simulink model "AC_gen_MGES"  (R2025a)
settings: Solver=VariableStepAuto  StartTime=0.0  StopTime=10.0  RelTol=1e-3
undefined symbols (not defined in the file): buses_lf, gen_static_params, Grid_op_MGES, Grid_op_SG, Matrix_flux_to_i, Ps_lf, Sb, SGs_nodes
(part 1 of 2)
settings Model: Creator=atomas  LastModifiedBy=atomas

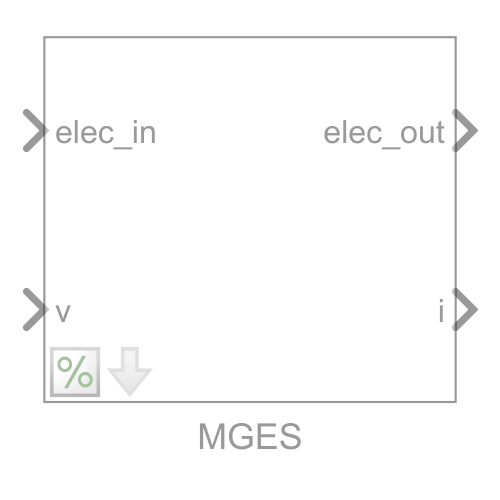
[thumbnail: Simulink's stored preview of the top-level diagram]
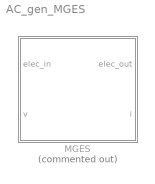
== system AC_gen_MGES ==
  MGES : Subsystem  Commented=on  mask(Synchronous machine){SGs_nodes=SGs_nodes, FBASE=50, D=0, H=3, Psimag_pu=0.8, Lssd_pu=0.1, Lssq_pu=0.1, Rs_pu=0.001, Lmd_pu=0.1, Lmq_pu=0.1, Rfd_pu=0.01, Lfd_pu=0.1, Rkd1_pu=1e6, Lkd1_pu=1e6, Rkd2_pu=1e6, Lkd2_pu=1e6, Rkq1_pu=1e6, Lkq1_pu=1e6, Rkq2_pu=1e6, Lkq2_pu=1e6, Rkq3_pu=1e6, Lkq3_pu=1e6, T_e=1, T_v=1, T_1=1, T_2=1, K_A=1, K_C=0, K_P=0, K_PR=1, K_IR=1, K_PM=1, K_IM=1, R_p=0.05, T_1g=1, T_2g=1, T_3=1, T_4=1, T_5=1, T_6=1, K_1=0, K_3=0, K_5=0, T_w1=1, T_w2=1, T_9=1, M=1, K_S1=0, T_1p=1, T_2p=1, T_3p=1, T_4p=1, T_7p=1, K_S2=1, K_S3=1}
      mask prompts: FBASE "Base frequency (Hz)"; D "Damping (pu)"; H "Inertia (s)"; Psimag_pu "Permanent flux (pu)"; Lssd_pu "Stator inductances (pu) Ld"; Lssq_pu "Stator inductances (pu) Lq"; Rs_pu "Stator resistances (pu)"; Lmd_pu "d-axis mutual inductance (pu)"; Lmq_pu "q-axis mutual inductance (pu)"; Rfd_pu "Excitation resistance (pu)"; Lfd_pu "Excitation inductance (pu)"; Rkd1_pu "d-axis damper resistance 1 (pu)"; Lkd1_pu "d-axis damper inductance 1 (pu)"; Rkd2_pu "d-axis damper resistance 2 (pu)"; Lkd2_pu "d-axis damper inductance 2 (pu)"; Rkq1_pu "q-axis damper resistance 1 (pu)"; Lkq1_pu "q-axis damper inductance 1 (pu)"; Rkq2_pu "q-axis damper resistance 2 (pu)"; Lkq2_pu "q-axis damper inductance 2 (pu)"; Rkq3_pu "q-axis damper resistance 3 (pu)"; Lkq3_pu "q-axis damper inductance 3 (pu)"; T_1p "T_1"
      mask help: Synchronous machine modelled in d-q reference frame.
      mask init:
      | mdlWks = get_param(bdroot,'ModelWorkspace'); % Get the model workspace
      | block_name = get_param(gcb,'Name');
      | try
      |     bvarname = get_param(get_param(get_param(...
      |         gcb, 'Parent'), 'Parent'), 'bvarname');
      |     block_buses = mdlWks.getVariable([bvarname block_name 's_buses']);
      | 	block_idx = mdlWks.getVariable([bvarname block_name '_idx']);
      |     block_toM = mdlWks.getVariable([bvarname block_name 's_toM']);
      |     fref = mdlWks.getVariable([bvarname 'fref']);
      |     block_fref = fref.(block_name);
      | catch ME % block in initialisation
      |     %errordlg(ME.message)
      |     try
      |         block_buses = 1:length(mdlWks.getVariable([block_name 's_buses']));
      | 	    block_idx = mdlWks.getVariable([block_name '_idx']);
      |         block_toM = mdlWks.getVariable([block_name 's_toM']);
      |         fref = mdlWks.getVariable('fref');
      | 	    block_fref = fref.(block_name);
      |     catch ME
      |         %errordlg(ME.message)
      |     end
      | end
      | 
      |     
      |     n = length(block_buses);
      |     Lbiginv = zeros(9*n,9*n);
      |     if isscalar(Lssd_pu)
      |         Lssd_pu = Lssd_pu*ones(1, n);
      |     end
      |     if isscalar(Lssq_pu)
      |         Lssq_pu = Lssq_pu*ones(1, n);
      |     end
      |     if isscalar(Lmd_pu)
      |         Lmd_pu = Lmd_pu*ones(1, n);
      |     end
      |     if isscalar(Lmq_pu)
      |         Lmq_pu = Lmq_pu*ones(1, n);
      |     end
      |     if isscalar(Lfd_pu)
      |         Lfd_pu = Lfd_pu*ones(1, n);
      |     end
      |     if isscalar(Lssd_pu)
      |         Lssd_pu = Lssd_pu*ones(1, n);
      |     end
      |     if isscalar(Lkd1_pu)
      |         Lkd1_pu = Lkd1_pu*ones(1, n);
      |     end
      |     if isscalar(Lkd2_pu)
      |         Lkd2_pu = Lkd2_pu*ones(1, n);
      |     end
      |     if isscalar(Lkq1_pu)
      |         Lkq1_pu = Lkq1_pu*ones(1, n);
      |     end
      |     if isscalar(Lkq2_pu)
      |         Lkq2_pu = Lkq2_pu*ones(1, n);
      |     end
      |     if isscalar(Lkq3_pu)
      |         Lkq3_pu = Lkq3_pu*ones(1, n);
      |     end
      |     for i=1:n
      |         j = 9*(i-1)+1;
      |         Ldq0 = [Lssd_pu(i), 0 0; 0, Lssq_pu(i), 0; 0, 0, 0.0001]; 
      |         Ladq0 = [Lmd_pu(i), Lmd_pu(i), Lmd_pu(i), 0 0 0; 0, 0, 0, Lmq_pu(i), Lmq_pu(i), Lmq_pu(i); zeros(1, 6)];
      |         Lk = [Lmd_pu(i)*ones(3,3), zeros(3,3); zeros(3,3), Lmq_pu(i)*ones(3,3)] +...
      |             diag([Lfd_pu(i), Lkd1_pu(i), Lkd2_pu(i), Lkq1_pu(i), Lkq2_pu(i), Lkq3_pu(i)]);
      |         L = [-Ldq0, Ladq0; -Ladq0', Lk];
      |         Lbiginv(j:(j+8), j:(j+8)) = inv(L);
      |     end
      | 
      |     if isscalar(K_C)
      |         K_C = K_C*ones(1, n);
      |     end
      |     if isscalar(K_P)
      |         K_P = K_P*ones(1, n);
      |     end
      |     if isscalar(T_1)
      |         T_1 = T_1*ones(1, n);
      |     end
      |     if isscalar(T_2)
      |         T_2 = T_2*ones(1, n);
      |     end
      mask Help: web([extractBefore(get_param(bdroot, 'filename'),gcs) 'Documentation/SM.html'])
      mask DialogControl Params Prompt: Parameters
      mask DialogControl AVR Prompt: AVR
      mask DialogControl Gov Prompt: Speed governor
      mask DialogControl PSS Prompt: Power system stabiliser

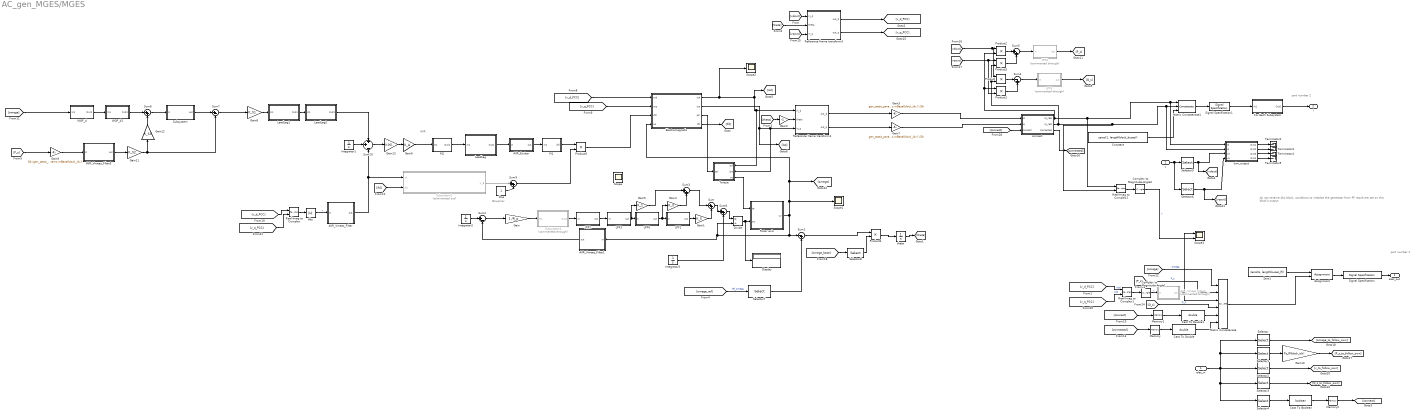
== system AC_gen_MGES/MGES ==
  note: AVR
  note: port number 2
  note: port number 1
  note: do not rename this block, conditions to initialise the generator from PF result are set on this block's output
  note: Governor
  elec_in : Inport
  v : Inport  Port=2
  AVR_Exciter : Subsystem  mask{T_s=T_e}
      mask prompts: T_s "Filter time constant"
  AVR_Vmeas_Filter : Subsystem  mask{T_r=T_v}
      mask prompts: T_r "Filter time constant"
  AVR_Vmeas_Filter1 : Subsystem  mask{T_r=0.01}
      mask prompts: T_r "Filter time constant"
  AVR_Vmeas_Filter2 : Subsystem  Commented=through  mask{T_r=0.01}
      mask prompts: T_r "Filter time constant"
      mask Display:
      | try
      |     dpoly(1, [T_r, 1])
      | catch
      | end
  AVR_Vmeas_Filter3 : Subsystem  mask{T_r=T_7p}
      mask prompts: T_r "Filter time constant"
  Abs : Abs  SaturateOnIntegerOverflow=off
  Assignment : Assignment  NumberOfDimensions=2  DiagnosticForDimensions=Warning  IndexOptions=Assign all,Index vector (dialog)  Indices=1,block_idx  OutputSizes=1,1
  Cast To Boolean : DataTypeConversion  OutDataTypeStr=boolean  SaturateOnIntegerOverflow=off  RndMeth=Floor
  Cast To Double : DataTypeConversion  OutDataTypeStr=double  SaturateOnIntegerOverflow=off  RndMeth=Floor
  Cast To Double1 : DataTypeConversion  OutDataTypeStr=double  SaturateOnIntegerOverflow=off  RndMeth=Floor
  Complex to Magnitude-Angle1 : ComplexToMagnitudeAngle  Output=Magnitude
  Complex to Magnitude-Angle2 : ComplexToMagnitudeAngle  Output=Magnitude
  Constant : Constant  Value=zeros(1, length(block_buses))  VectorParams1D=off
  Display : Display
  Divide : Product  Inputs=*/
  Electromagnetic : Subsystem  Variant=on  VariantControlMode=label  LabelModeActiveChoice=order 8
  For Each Subsystem : Subsystem  TreatAsAtomicUnit=on
  Gain : Gain  Gain=1./R_p
  Gain1 : Gain  Gain=K_5
  Gain10 : Gain  Gain=Ps_lf(block_idx)
  Gain11 : Gain  Gain=K_S2
  Gain12 : Gain  Gain=K_S3
  Gain13 : Gain  Gain=0.001
  Gain2 : Gain  Gain=-1
  Gain3 : Gain  Gain=gen_static_params.mBase(block_idx)'./Sb
  Gain4 : Gain  Gain=K_3
  Gain5 : Gain  Gain=K_1
  Gain6 : Gain  Gain=K_A
  Gain7 : Gain  Gain=gen_static_params.mBase(block_idx)'./Sb
  Gain8 : Gain  Gain=K_S1
  Gain9 : Gain  Gain=Sb./gen_static_params.mBase(block_idx)'
  Integrator1 : Integrator  InitialCondition=Grid_op_MGES.op.States(13).x'
  Integrator2 : Integrator  InitialCondition=Grid_op_MGES.op.States(14).x'
  Integrator3 : Integrator  InitialCondition=Grid_op_MGES.op.States(15).x'
  LPF1 : Subsystem  mask{T_s=T_6}
      mask prompts: T_s "Filter time constant"
  LPF2 : Subsystem  mask{T_s=T_3}
      mask prompts: T_s "Filter time constant"
  LPF3 : Subsystem  mask{T_s=T_4}
      mask prompts: T_s "Filter time constant"
  LPF4 : Subsystem  Commented=through  mask{T_s=0.01}
      mask prompts: T_s "Filter time constant"
      mask Display:
      | try
      |     dpoly(1, [T_s, 1])
      | catch
      | end
  LPF5 : Subsystem  Commented=through  mask{T_s=0.01}
      mask prompts: T_s "Filter time constant"
      mask Display:
      | try
      |     dpoly(1, [T_s, 1])
      | catch
      | end
  LPF6 : Subsystem  mask{T_s=T_5}
      mask prompts: T_s "Filter time constant"
  LeadLag : Subsystem
  LeadLag1 : Subsystem  mask{T_2=T_1p, T_1=T_2p}
      mask help:
      | Transfer function:
      |
      |   1 + sT_2
      | ---------------
      |   1 + sT_1
  LeadLag2 : Subsystem  mask{T_2=T_3p, T_1=T_4p}
      mask help:
      | Transfer function:
      |
      |   1 + sT_2
      | ---------------
      |   1 + sT_1
  Matrix Concatenate : Concatenate  NumInputs=6  Mode=Multidimensional array
  Matrix Concatenate1 : Concatenate  NumInputs=3  Mode=Multidimensional array
  Memory : Memory  InitialCondition=1
  Memory1 : Memory  InitialCondition=1
  Memory2 : Memory  InitialCondition=1
  One : Constant  OutDataTypeStr=Inherit: Inherit via back propagation
  PI1 : Subsystem
  PI2 : Subsystem
  Product{,1..5} (6 alike) : Product
  Real-Imag to Complex : RealImagToComplex
  Real-Imag to Complex1 : RealImagToComplex
  Real-Imag to Complex2 : RealImagToComplex
  Reference frame transform1 : Subsystem
  Reference frame transform3 : Subsystem
  Rotor axis : Subsystem
  Scope : Scope
      settings: ActiveDisplayYMinimum=-1  ActiveDisplayYMaximum=1  DataLoggingVariableName=ScopeData13
  Scope1 : Scope
      settings: ActiveDisplayYMinimum=-0.058141408811601208  ActiveDisplayYMaximum=2.1702525958532117  DataLoggingVariableName=ScopeData3
  Scope2 : Scope
      settings: ActiveDisplayYMinimum=-0.402690614368146  ActiveDisplayYMaximum=1.3038964261892889  DataLoggingVariableName=ScopeData9
  Scope3 : Scope  NumInputPorts=2
      settings: ActiveDisplayYMinimum=0.29123  ActiveDisplayYMaximum=1.9416  DataLoggingVariableName=ScopeData3
  Selector : Selector  NumberOfDimensions=2  InputPortWidth=3  IndexOptions=Index vector (dialog),Index vector (dialog)  Indices=1,block_idx  OutputSizes=1,1
  Selector1 : Selector  NumberOfDimensions=2  InputPortWidth=3  IndexOptions=Index vector (dialog),Index vector (dialog)  Indices=2,block_idx  OutputSizes=1,1
  Selector2 : Selector  NumberOfDimensions=2  InputPortWidth=3  IndexOptions=Index vector (dialog),Index vector (dialog)  Indices=3,block_idx  OutputSizes=1,1
  Selector3 : Selector  NumberOfDimensions=2  InputPortWidth=3  IndexOptions=Index vector (dialog),Index vector (dialog)  Indices=4,block_idx  OutputSizes=1,1
  Selector4 : Selector  NumberOfDimensions=2  InputPortWidth=3  IndexOptions=Index vector (dialog),Index vector (dialog)  Indices=5,block_idx  OutputSizes=1,1
  Selector5 : Selector  NumberOfDimensions=2  InputPortWidth=3  IndexOptions=Index vector (dialog),Index vector (dialog)  Indices=1,block_buses  OutputSizes=1,1
  Selector6 : Selector  NumberOfDimensions=2  InputPortWidth=3  IndexOptions=Index vector (dialog),Index vector (dialog)  Indices=2,block_buses  OutputSizes=1,1
  Selector7 : Selector  InputPortWidth=length(fref.ref_units)  IndexOptions=Index vector (dialog)  Indices=block_fref  OutputSizes=1
  Selector8 : Selector  InputPortWidth=length(fref.ref_units)  IndexOptions=Index vector (dialog)  Indices=block_fref  OutputSizes=1
  Signal Specification : SignalSpecification  Dimensions=[6 length(buses_lf)]
  Signal Specification1 : SignalSpecification  Dimensions=[3 length(block_buses)]
  Subsystem : Subsystem
  Subsystem1 : Subsystem  Commented=on  mask{K_P=K_P}
      mask init:
      | if all(K_P == 0)
      |         set_param(gcb, 'Commented', 'on')
      |     else
      |         set_param(gcb, 'Commented', 'off')
      |     end
  Subsystem4 : Subsystem  Commented=through  mask{T_2=T_2, T_1=T_1}
      mask help:
      | Transfer function:
      |
      |   1 + sT_2
      | ---------------
      |   1 + sT_1
  Sum{,3,5..6,8..9} (6 alike) : Sum  Inputs=|++
  Sum1 : Sum  Inputs=|-+
  Sum10 : Sum  Inputs=+|+|-
  Sum2 : Sum  Inputs=|+-
  Sum4 : Sum  Inputs=|-+
  Sum7 : Sum  Inputs=|+-
  Terminator{2..5} (4 alike) : Terminator
  Torque : Subsystem
      settings: PortSchema="{\"entries\":[{\"content\":{\"sides\":[{\"content\":{\"connectorIds\":[\"In1\"]},\"type\":\"ConnectorPlacement.EquallySpacedRectSide\",\"uuid\":\"b7abd3bc-22dd-4669-aa40-98bc76884565\"},{\"content\":{\"connectorIds\":[\"In2\",\"In3\",\"Out1\"],\"side\":\"RIGHT\"},\"type\":\"ConnectorPlacement.EquallySpacedRectSide\",\"uuid\":\"e9abb552-b46d-48ed-aa1f-0e9dac604fea\"},{\"content\":{\"connectorIds\":[],\"side\":\"TOP\"},\"type\":\"ConnectorPlacement.EquallySpacedRectSide\",\"uuid\":\"4b14997d-8f32-4cfb-8a1b-18cffb093d28\"}]},\"type\":\"ConnectorPlacement.EquallySpacedConnector\",\"uuid\":\"d6624493-e930-4f0d-8cbe-17f96cb72edc\"}],\"packageUris\":[\"http://schema.mathworks.com/mf0/Connector/R2020b\"],\"version\":\"1.0\"}"
  WOF_d : Subsystem
  WOF_d1 : Subsystem
  Zero1 : Constant  Value=zeros(6, length(buses_lf))  VectorParams1D=off  OutDataTypeStr=Inherit: Inherit via back propagation
  connect : Subsystem
  theta : Integrator  InitialCondition=Grid_op_MGES.op.States(33).x'  UpperSaturationLimit=2*pi  LowerSaturationLimit=0
  trim_output : Subsystem
  elec_out : Outport
  i : Outport  Port=2
  wires:
  One/1 -> Sum9/2
  Sum9/1 -> Product5/2
  Subsystem1/1(V_B) -> Sum9/1
  Product5/1 -> Electromagnetic/3(vfd)
  Divide/1 -> Rotor axis/2(tm), Display/1
  LeadLag2/1(Out1) -> Sum10/1
  Gain9/1 -> AVR_Vmeas_Filter3/1(in)
  Integrator3/1 -> Sum8/2
  Sum8/1 -> Divide/1
  Sum/1 -> Sum8/1
  Gain13/1 -> Gain6/1
  Sum10/1 -> Gain13/1
  Torque/1(te) -> Rotor axis/1(te)
  Integrator2/1 -> Sum2/1
  [P_s] -> Gain9/1
  AVR_Vmeas_Filter3/1(out) -> Gain11/1
  Gain11/1 -> Gain12/1, Sum7/2
  Gain12/1 -> Sum6/2
  Sum7/1 -> Gain8/1
  Subsystem/1(out) -> Sum7/1
  Sum6/1 -> Subsystem/1(in)
  WOF_d1/1(Out1) -> Sum6/1
  [omega] -> WOF_d/1(In1)
  LeadLag1/1(Out1) -> LeadLag2/1(In1)
  Gain8/1 -> LeadLag1/1(In1)
  WOF_d/1(Out1) -> WOF_d1/1(In1)
  Gain7/1 -> connect/2(iq)
  Gain3/1 -> connect/1(id)
  Gain5/1 -> Sum3/1
  Gain4/1 -> Sum3/2
  Sum3/1 -> Sum/1
  Rotor axis/1(wr) -> AVR_Vmeas_Filter1/1(in), Divide/2, Sum1/1, Scope1/1, [omega], Electromagnetic/4(ws)
  Gain1/1 -> Sum/2
  LPF1/1(out) -> Gain1/1
  LPF3/1(out) -> LPF6/1(in), Gain5/1
  PI1/1(vfd) -> Product5/1
  [ifd] -> Subsystem1/2(ifd)
  AVR_Exciter/1(out) -> PI1/1(In1)
  PI2/1(Out1) -> LeadLag/1(In1)
  Electromagnetic/4(ifd) -> [ifd]
  Electromagnetic/3(psi) -> Torque/1(psi)
  [v_q_PCC] -> Electromagnetic/2(vsq)
  [v_d_PCC] -> Electromagnetic/1(vsd)
  Electromagnetic/1(isd) -> [isd], Torque/2(isd), Reference frame transform1/1(in_d), Scope2/1
  Electromagnetic/2(isq) -> Reference frame transform1/3(in_q), Torque/3(isq), [isq]
  Complex to Magnitude-Angle2/1 -> Scope3/2  "v"
  Real-Imag to Complex2/1 -> Complex to Magnitude-Angle2/1
  AVR_Vmeas_Filter2/1(out) -> Scope3/1, Matrix Concatenate/3
  AVR_Vmeas_Filter1/1(out) -> Sum2/2
  Real-Imag to Complex/1 -> Abs/1
  [v_q_PCC] -> Real-Imag to Complex/2
  Abs/1 -> AVR_Vmeas_Filter/1(in)  "v"
  [v_d_PCC] -> Real-Imag to Complex/1
  LeadLag/1(Out1) -> AVR_Exciter/1(in)
  AVR_Vmeas_Filter/1(out) -> Subsystem1/1(vt), Sum10/3
  Gain6/1 -> PI2/1(In1)
  Integrator1/1 -> Sum10/2
  Sum2/1 -> Gain/1
  Gain/1 -> Subsystem4/1(In1)
  Sum1/1 -> Product4/1
  Product4/1 -> theta/1
  [omega_base] -> Selector8/1
  Selector8/1 -> Product4/2
  Selector7/1 -> Sum1/2
  Memory2/1 -> [connect]
  Memory1/1 -> Cast To Double1/1
  Gain10/1 -> [P_s_to_follow_own]
  Memory/1 -> Cast To Double/1
  Reference frame transform3/2(out_q) -> [v_q_PCC]
  Reference frame transform3/1(out_d) -> [v_d_PCC]
  [vdout] -> Reference frame transform3/1(in_d)
  [vqout] -> Reference frame transform3/3(in_q)
  Selector6/1 -> trim_output/4(vq), [vqout]
  Selector5/1 -> trim_output/3(vd), [vdout]
  v/1 -> Selector5/1, Selector6/1
  trim_output/2(Out2) -> Terminator3/1
  trim_output/4(Out4) -> Terminator5/1
  trim_output/1(Out1) -> Terminator2/1
  trim_output/3(Out3) -> Terminator4/1
  connect/2(iq_real) -> Matrix Concatenate1/2, trim_output/2(iq), Real-Imag to Complex2/2, Product/2, Product3/2
  For Each Subsystem/1(Out1) -> i/1
  Constant/1 -> Matrix Concatenate1/3
  Signal Specification1/1 -> For Each Subsystem/1(In1)
  Matrix Concatenate1/1 -> Signal Specification1/1
  Matrix Concatenate/1 -> Assignment/2
  Assignment/1 -> Signal Specification/1
  elec_in/1 -> Selector/1, Selector1/1, Selector2/1, Selector3/1, Selector4/1
  Signal Specification/1 -> elec_out/1
  Zero1/1 -> Assignment/1
  Cast To Boolean/1 -> Memory2/1
  Selector4/1 -> Cast To Boolean/1
  connect/1(id_real) -> Product2/2, Product1/1, Matrix Concatenate1/1, trim_output/1(id), Real-Imag to Complex2/1
  [connect] -> connect/3(connect)
  connect/3(connected) -> [connected]
  [v_q_PCC] -> Real-Imag to Complex1/2  "voq"
  [v_d_PCC] -> Real-Imag to Complex1/1  "vod"
  [vqout] -> Product1/2, Product3/1
  [vdout] -> Product2/1, Product/1
  Real-Imag to Complex1/1 -> Complex to Magnitude-Angle1/1
  Cast To Double/1 -> Matrix Concatenate/6
  Cast To Double1/1 -> Matrix Concatenate/5
  [connected] -> Memory/1
  [connect] -> Memory1/1
  Selector2/1 -> [v_to_follow_own]
  Selector1/1 -> Gain10/1
  Selector/1 -> [omega_to_follow_own]
  Selector3/1 -> [Q_s_to_follow_own]
  [Q_s] -> Matrix Concatenate/4  "Q_s"
  Complex to Magnitude-Angle1/1 -> AVR_Vmeas_Filter2/1(in)  "v"
  [omega] -> Matrix Concatenate/1  "omega"
  [P_s] -> Matrix Concatenate/2  "P_s"
  LPF4/1(out) -> [P_s]
  Subsystem4/1(Out1) -> LPF2/1(in)
  Reference frame transform1/1(out_d) -> Gain3/1
  Product2/1 -> Sum5/1
  [omega_ref] -> Selector7/1  "ref_omega"
  Product3/1 -> Sum5/2
  Sum5/1 -> LPF4/1(in)
  Sum4/1 -> LPF5/1(in)
  LPF2/1(out) -> LPF3/1(in)
  [theta] -> Gain2/1
  LPF6/1(out) -> LPF1/1(in), Gain4/1
  [theta] -> Reference frame transform3/2(theta)
  Gain2/1 -> Reference frame transform1/2(theta)
  theta/1 -> [theta]
  Product1/1 -> Sum4/2
  Product/1 -> Sum4/1
  Reference frame transform1/2(out_q) -> Gain7/1
  LPF5/1(out) -> [Q_s]

== system AC_gen_MGES/MGES/AVR_Exciter ==
  in : Inport
  Gain : Gain  Gain=1./T_s
  Sum4 : Sum  Inputs=|+-
  x_a : Integrator  InitialCondition=Grid_op_MGES.op.States(1).x'
  out : Outport
  wires:
  x_a/1 -> Sum4/2, out/1
  in/1 -> Sum4/1
  Sum4/1 -> Gain/1
  Gain/1 -> x_a/1

== system AC_gen_MGES/MGES/AVR_Vmeas_Filter ==
  in : Inport
  Gain : Gain  Gain=1./T_r
  Sum4 : Sum  Inputs=|+-
  x_a : Integrator  InitialCondition=Grid_op_MGES.op.States(2).x'
  out : Outport
  wires:
  x_a/1 -> Sum4/2, out/1
  in/1 -> Sum4/1
  Sum4/1 -> Gain/1
  Gain/1 -> x_a/1

== system AC_gen_MGES/MGES/AVR_Vmeas_Filter1 ==
  in : Inport
  Gain : Gain  Gain=1/T_r
  Sum4 : Sum  Inputs=|+-
  x_a : Integrator  InitialConditionSource=external  InitialCondition=Grid_op_MGES.op.States(3).x'
  out : Outport
  wires:
  Gain/1 -> x_a/1
  Sum4/1 -> Gain/1
  in/1 -> Sum4/1, x_a/2
  x_a/1 -> out/1, Sum4/2

== system AC_gen_MGES/MGES/AVR_Vmeas_Filter2 ==
  in : Inport
  Gain : Gain  Gain=1/T_r
  Sum4 : Sum  Inputs=|+-
  x_a : Integrator  InitialCondition=Grid_op_SG.op.States(5).x'
  out : Outport
  wires:
  x_a/1 -> Sum4/2, out/1
  in/1 -> Sum4/1
  Sum4/1 -> Gain/1
  Gain/1 -> x_a/1

== system AC_gen_MGES/MGES/AVR_Vmeas_Filter3 ==
  in : Inport
  Gain : Gain  Gain=1./T_r
  Sum4 : Sum  Inputs=|+-
  x_a : Integrator  InitialCondition=Grid_op_MGES.op.States(4).x'
  out : Outport
  wires:
  Gain/1 -> x_a/1
  Sum4/1 -> Gain/1
  in/1 -> Sum4/1
  x_a/1 -> out/1, Sum4/2

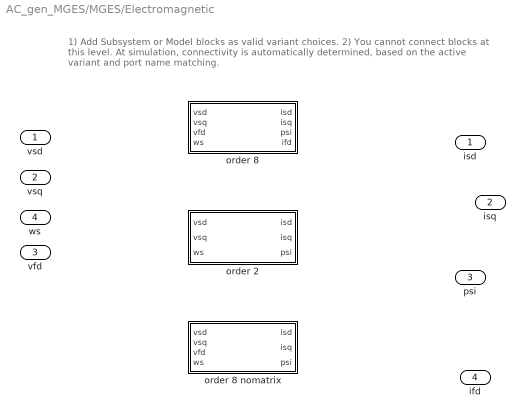
== system AC_gen_MGES/MGES/Electromagnetic ==
  note: 1) Add Subsystem or Model blocks as valid variant choices.
      | 2) You cannot connect blocks at this level. At simulation, connectivity is automatically
      | determined, based on the active variant and port name matching.
  vsd : Inport
  vsq : Inport  Port=2
  vfd : Inport  Port=3
  ws : Inport  Port=4
  order 2 : Subsystem  VariantControl=order 2
  order 8 : Subsystem  VariantControl=order 8
  order 8 nomatrix : Subsystem  VariantControl=order 1  mask{Lssd_pu=Lssd_pu, Lssq_pu=Lssq_pu, Lmd_pu=Lmd_pu, Lmq_pu=Lmq_pu, Lfd_pu=Lfd_pu, Lkd1_pu=Lkd1_pu, Lkd2_pu=Lkd2_pu, Lkq1_pu=Lkq1_pu, Lkq2_pu=Lkq2_pu, Lkq3_pu=Lkq3_pu}
      mask init:
      | for i=1:length(Lssd_pu)
      |         Lssd = Lssd_pu;
      |         Lssq = Lssq_pu;
      |         Lmd = Lmd_pu;
      |         Lmq = Lmq_pu;
      |         Lfd = Lfd_pu;
      |         Lkd1 = Lkd1_pu;
      |         Lkd2 = Lkd2_pu;
      |         Lkq1 = Lkq1_pu;
      |         Lkq2 = Lkq2_pu;
      |         Lkq3 = Lkq3_pu;
      |         Matrix_flux_to_i(:,:,i) = [(0 - (Lfd(i)*Lmd(i)^2 + Lkd2(i)*Lmd(i)^2 - Lmd(i)^3 - Lfd(i)*Lkd1(i)*Lkd2(i))/(2*Lmd(i)^4 - Lkd1(i)*Lmd(i)^3 - 2*Lkd2(i)*Lmd(i)^3 - Lmd(i)^3*Lssd(i) - 2*Lfd(i)*Lmd(i)^3 + Lfd(i)*Lkd1(i)*Lmd(i)^2 + Lfd(i)*Lkd2(i)*Lmd(i)^2 + Lkd1(i)*Lkd2(i)*Lmd(i)^2 + Lfd(i)*Lmd(i)^2*Lssd(i) + Lkd2(i)*Lmd(i)^2*Lssd(i) - Lfd(i)*Lkd1(i)*Lkd2(i)*Lssd(i))),  + 0,  + (0 + (Lkd1(i)*Lmd(i)^2 + Lkd2(i)*Lmd(i)^2 - Lmd(i)^3 - Lkd1(i)*Lkd2(i)*Lmd(i))/(2*Lmd(i)^4 - Lkd1(i)*Lmd(i)^3 - 2*Lkd2(i)*Lmd(i)^3 - Lmd(i)^3*Lssd(i) - 2*Lfd(i)*Lmd(i)^3 + Lfd(i)*Lkd1(i)*Lmd(i)^2 + Lfd(i)*Lkd2(i)*Lmd(i)^2 + Lkd1(i)*Lkd2(i)*Lmd(i)^2 + Lfd(i)*Lmd(i)^2*Lssd(i) + Lkd2(i)*Lmd(i)^2*Lssd(i) - Lfd(i)*Lkd1(i)*Lkd2(i)*Lssd(i))),  + (0 + (Lfd(i)*Lmd(i)^2 + Lkd2(i)*Lmd(i)^2 - Lmd(i)^3 - Lfd(i)*Lkd2(i)*Lmd(i))/(2*Lmd(i)^4 - Lkd1(i)*Lmd(i)^3 - 2*Lkd2(i)*Lmd(i)^3 - Lmd(i)^3*Lssd(i) - 2*Lfd(i)*Lmd(i)^3 + Lfd(i)*Lkd1(i)*Lmd(i)^2 + Lfd(i)*Lkd2(i)*Lmd(i)^2 + Lkd1(i)*Lkd2(i)*Lmd(i)^2 + Lfd(i)*Lmd(i)^2*Lssd(i) + Lkd2(i)*Lmd(i)^2*Lssd(i) - Lfd(i)*Lkd1(i)*Lkd2(i)*Lssd(i))),  + (0 + (Lfd(i)*Lmd(i)^2 - Lfd(i)*Lkd1(i)*Lmd(i))/(2*Lmd(i)^4 - Lkd1(i)*Lmd(i)^3 - 2*Lkd2(i)*Lmd(i)^3 - Lmd(i)^3*Lssd(i) - 2*Lfd(i)*Lmd(i)^3 + Lfd(i)*Lkd1(i)*Lmd(i)^2 + Lfd(i)*Lkd2(i)*Lmd(i)^2 + Lkd1(i)*Lkd2(i)*Lmd(i)^2 + Lfd(i)*Lmd(i)^2*Lssd(i) + Lkd2(i)*Lmd(i)^2*Lssd(i) - Lfd(i)*Lkd1(i)*Lkd2(i)*Lssd(i))),  + 0,  + 0,  + 0, ; 0,  + (0 - (Lkq1(i)*Lmq(i)^2 + Lkq2(i)*Lmq(i)^2 + Lkq3(i)*Lmq(i)^2 - 2*Lmq(i)^3 - Lkq1(i)*Lkq2(i)*Lkq3(i))/(3*Lmq(i)^4 - 2*Lkq2(i)*Lmq(i)^3 - 2*Lkq3(i)*Lmq(i)^3 - 2*Lmq(i)^3*Lssq(i) - 2*Lkq1(i)*Lmq(i)^3 + Lkq1(i)*Lkq2(i)*Lmq(i)^2 + Lkq1(i)*Lkq3(i)*Lmq(i)^2 + Lkq2(i)*Lkq3(i)*Lmq(i)^2 + Lkq1(i)*Lmq(i)^2*Lssq(i) + Lkq2(i)*Lmq(i)^2*Lssq(i) + Lkq3(i)*Lmq(i)^2*Lssq(i) - Lkq1(i)*Lkq2(i)*Lkq3(i)*Lssq(i))),  + 0,  + 0,  + 0,  + (0 - (3*Lmq(i)^3 - 2*Lkq2(i)*Lmq(i)^2 - 2*Lkq3(i)*Lmq(i)^2 - 2*Lkq1(i)*Lmq(i)^2 + Lkq1(i)*Lkq2(i)*Lmq(i) + Lkq1(i)*Lkq3(i)*Lmq(i) + Lkq2(i)*Lkq3(i)*Lmq(i))/(3*Lmq(i)^4 - 2*Lkq2(i)*Lmq(i)^3 - 2*Lkq3(i)*Lmq(i)^3 - 2*Lmq(i)^3*Lssq(i) - 2*Lkq1(i)*Lmq(i)^3 + Lkq1(i)*Lkq2(i)*Lmq(i)^2 + Lkq1(i)*Lkq3(i)*Lmq(i)^2 + Lkq2(i)*Lkq3(i)*Lmq(i)^2 + Lkq1(i)*Lmq(i)^2*Lssq(i) + Lkq2(i)*Lmq(i)^2*Lssq(i) + Lkq3(i)*Lmq(i)^2*Lssq(i) - Lkq1(i)*Lkq2(i)*Lkq3(i)*Lssq(i))),  + 0,  + 0, ; (0 - (Lkd2(i)*Lmd(i)^2 - Lkd1(i)*Lkd2(i)*Lmd(i))/(2*Lmd(i)^4 - Lkd1(i)*Lmd(i)^3 - 2*Lkd2(i)*Lmd(i)^3 - Lmd(i)^3*Lssd(i) - 2*Lfd(i)*Lmd(i)^3 + Lfd(i)*Lkd1(i)*Lmd(i)^2 + Lfd(i)*Lkd2(i)*Lmd(i)^2 + Lkd1(i)*Lkd2(i)*Lmd(i)^2 + Lfd(i)*Lmd(i)^2*Lssd(i) + Lkd2(i)*Lmd(i)^2*Lssd(i) - Lfd(i)*Lkd1(i)*Lkd2(i)*Lssd(i))),  + 0,  + (0 + (Lkd1(i)*Lmd(i)^2 + Lkd2(i)*Lmd(i)^2 + Lmd(i)^2*Lssd(i) - 2*Lmd(i)^3 - Lkd1(i)*Lkd2(i)*Lssd(i))/(2*Lmd(i)^4 - Lkd1(i)*Lmd(i)^3 - 2*Lkd2(i)*Lmd(i)^3 - Lmd(i)^3*Lssd(i) - 2*Lfd(i)*Lmd(i)^3 + Lfd(i)*Lkd1(i)*Lmd(i)^2 + Lfd(i)*Lkd2(i)*Lmd(i)^2 + Lkd1(i)*Lkd2(i)*Lmd(i)^2 + Lfd(i)*Lmd(i)^2*Lssd(i) + Lkd2(i)*Lmd(i)^2*Lssd(i) - Lfd(i)*Lkd1(i)*Lkd2(i)*Lssd(i))),  + (0 - (Lkd2(i)*Lmd(i)^2 - Lkd2(i)*Lssd(i)*Lmd(i))/(2*Lmd(i)^4 - Lkd1(i)*Lmd(i)^3 - 2*Lkd2(i)*Lmd(i)^3 - Lmd(i)^3*Lssd(i) - 2*Lfd(i)*Lmd(i)^3 + Lfd(i)*Lkd1(i)*Lmd(i)^2 + Lfd(i)*Lkd2(i)*Lmd(i)^2 + Lkd1(i)*Lkd2(i)*Lmd(i)^2 + Lfd(i)*Lmd(i)^2*Lssd(i) + Lkd2(i)*Lmd(i)^2*Lssd(i) - Lfd(i)*Lkd1(i)*Lkd2(i)*Lssd(i))),  + (0 - (Lkd1(i)*Lmd(i)^2 + Lmd(i)^2*Lssd(i) - 2*Lmd(i)^3)/(2*Lmd(i)^4 - Lkd1(i)*Lmd(i)^3 - 2*Lkd2(i)*Lmd(i)^3 - Lmd(i)^3*Lssd(i) - 2*Lfd(i)*Lmd(i)^3 + Lfd(i)*Lkd1(i)*Lmd(i)^2 + Lfd(i)*Lkd2(i)*Lmd(i)^2 + Lkd1(i)*Lkd2(i)*Lmd(i)^2 + Lfd(i)*Lmd(i)^2*Lssd(i) + Lkd2(i)*Lmd(i)^2*Lssd(i) - Lfd(i)*Lkd1(i)*Lkd2(i)*Lssd(i))),  + 0,  + 0,  + 0, ; (0 - (Lfd(i)*Lmd(i)^2 + Lkd2(i)*Lmd(i)^2 - Lmd(i)^3 - Lfd(i)*Lkd2(i)*Lmd(i))/(2*Lmd(i)^4 - Lkd1(i)*Lmd(i)^3 - 2*Lkd2(i)*Lmd(i)^3 - Lmd(i)^3*Lssd(i) - 2*Lfd(i)*Lmd(i)^3 + Lfd(i)*Lkd1(i)*Lmd(i)^2 + Lfd(i)*Lkd2(i)*Lmd(i)^2 + Lkd1(i)*Lkd2(i)*Lmd(i)^2 + Lfd(i)*Lmd(i)^2*Lssd(i) + Lkd2(i)*Lmd(i)^2*Lssd(i) - Lfd(i)*Lkd1(i)*Lkd2(i)*Lssd(i))),  + 0,  + (0 - (Lkd2(i)*Lmd(i)^2 + Lmd(i)^2*Lssd(i) - Lmd(i)^3 - Lkd2(i)*Lmd(i)*Lssd(i))/(2*Lmd(i)^4 - Lkd1(i)*Lmd(i)^3 - 2*Lkd2(i)*Lmd(i)^3 - Lmd(i)^3*Lssd(i) - 2*Lfd(i)*Lmd(i)^3 + Lfd(i)*Lkd1(i)*Lmd(i)^2 + Lfd(i)*Lkd2(i)*Lmd(i)^2 + Lkd1(i)*Lkd2(i)*Lmd(i)^2 + Lfd(i)*Lmd(i)^2*Lssd(i) + Lkd2(i)*Lmd(i)^2*Lssd(i) - Lfd(i)*Lkd1(i)*Lkd2(i)*Lssd(i))),  + (0 + (Lfd(i)*Lmd(i)^2 + Lkd2(i)*Lmd(i)^2 - Lmd(i)^3 - Lfd(i)*Lkd2(i)*Lssd(i))/(2*Lmd(i)^4 - Lkd1(i)*Lmd(i)^3 - 2*Lkd2(i)*Lmd(i)^3 - Lmd(i)^3*Lssd(i) - 2*Lfd(i)*Lmd(i)^3 + Lfd(i)*Lkd1(i)*Lmd(i)^2 + Lfd(i)*Lkd2(i)*Lmd(i)^2 + Lkd1(i)*Lkd2(i)*Lmd(i)^2 + Lfd(i)*Lmd(i)^2*Lssd(i) + Lkd2(i)*Lmd(i)^2*Lssd(i) - Lfd(i)*Lkd1(i)*Lkd2(i)*Lssd(i))),  + (0 - (Lfd(i)*Lmd(i)^2 - Lfd(i)*Lssd(i)*Lmd(i))/(2*Lmd(i)^4 - Lkd1(i)*Lmd(i)^3 - 2*Lkd2(i)*Lmd(i)^3 - Lmd(i)^3*Lssd(i) - 2*Lfd(i)*Lmd(i)^3 + Lfd(i)*Lkd1(i)*Lmd(i)^2 + Lfd(i)*Lkd2(i)*Lmd(i)^2 + Lkd1(i)*Lkd2(i)*Lmd(i)^2 + Lfd(i)*Lmd(i)^2*Lssd(i) + Lkd2(i)*Lmd(i)^2*Lssd(i) - Lfd(i)*Lkd1(i)*Lkd2(i)*Lssd(i))),  + 0,  + 0,  + 0, ; (0 - (Lfd(i)*Lmd(i)^2 + Lkd1(i)*Lmd(i)^2 - Lmd(i)^3 - Lfd(i)*Lkd1(i)*Lmd(i))/(2*Lmd(i)^4 - Lkd1(i)*Lmd(i)^3 - 2*Lkd2(i)*Lmd(i)^3 - Lmd(i)^3*Lssd(i) - 2*Lfd(i)*Lmd(i)^3 + Lfd(i)*Lkd1(i)*Lmd(i)^2 + Lfd(i)*Lkd2(i)*Lmd(i)^2 + Lkd1(i)*Lkd2(i)*Lmd(i)^2 + Lfd(i)*Lmd(i)^2*Lssd(i) + Lkd2(i)*Lmd(i)^2*Lssd(i) - Lfd(i)*Lkd1(i)*Lkd2(i)*Lssd(i))),  + 0,  + (0 - (Lkd1(i)*Lmd(i)^2 + Lmd(i)^2*Lssd(i) - Lmd(i)^3 - Lkd1(i)*Lmd(i)*Lssd(i))/(2*Lmd(i)^4 - Lkd1(i)*Lmd(i)^3 - 2*Lkd2(i)*Lmd(i)^3 - Lmd(i)^3*Lssd(i) - 2*Lfd(i)*Lmd(i)^3 + Lfd(i)*Lkd1(i)*Lmd(i)^2 + Lfd(i)*Lkd2(i)*Lmd(i)^2 + Lkd1(i)*Lkd2(i)*Lmd(i)^2 + Lfd(i)*Lmd(i)^2*Lssd(i) + Lkd2(i)*Lmd(i)^2*Lssd(i) - Lfd(i)*Lkd1(i)*Lkd2(i)*Lssd(i))),  + (0 - (Lfd(i)*Lmd(i)^2 + Lmd(i)^2*Lssd(i) - Lmd(i)^3 - Lfd(i)*Lmd(i)*Lssd(i))/(2*Lmd(i)^4 - Lkd1(i)*Lmd(i)^3 - 2*Lkd2(i)*Lmd(i)^3 - Lmd(i)^3*Lssd(i) - 2*Lfd(i)*Lmd(i)^3 + Lfd(i)*Lkd1(i)*Lmd(i)^2 + Lfd(i)*Lkd2(i)*Lmd(i)^2 + Lkd1(i)*Lkd2(i)*Lmd(i)^2 + Lfd(i)*Lmd(i)^2*Lssd(i) + Lkd2(i)*Lmd(i)^2*Lssd(i) - Lfd(i)*Lkd1(i)*Lkd2(i)*Lssd(i))),  + (0 + (Lfd(i)*Lmd(i)^2 + Lkd1(i)*Lmd(i)^2 + Lmd(i)^2*Lssd(i) - 2*Lmd(i)^3 - Lfd(i)*Lkd1(i)*Lssd(i))/(2*Lmd(i)^4 - Lkd1(i)*Lmd(i)^3 - 2*Lkd2(i)*Lmd(i)^3 - Lmd(i)^3*Lssd(i) - 2*Lfd(i)*Lmd(i)^3 + Lfd(i)*Lkd1(i)*Lmd(i)^2 + Lfd(i)*Lkd2(i)*Lmd(i)^2 + Lkd1(i)*Lkd2(i)*Lmd(i)^2 + Lfd(i)*Lmd(i)^2*Lssd(i) + Lkd2(i)*Lmd(i)^2*Lssd(i) - Lfd(i)*Lkd1(i)*Lkd2(i)*Lssd(i))),  + 0,  + 0,  + 0, ; 0,  + (0 - (Lkq2(i)*Lmq(i)^2 + Lkq3(i)*Lmq(i)^2 - Lmq(i)^3 - Lkq2(i)*Lkq3(i)*Lmq(i))/(3*Lmq(i)^4 - 2*Lkq2(i)*Lmq(i)^3 - 2*Lkq3(i)*Lmq(i)^3 - 2*Lmq(i)^3*Lssq(i) - 2*Lkq1(i)*Lmq(i)^3 + Lkq1(i)*Lkq2(i)*Lmq(i)^2 + Lkq1(i)*Lkq3(i)*Lmq(i)^2 + Lkq2(i)*Lkq3(i)*Lmq(i)^2 + Lkq1(i)*Lmq(i)^2*Lssq(i) + Lkq2(i)*Lmq(i)^2*Lssq(i) + Lkq3(i)*Lmq(i)^2*Lssq(i) - Lkq1(i)*Lkq2(i)*Lkq3(i)*Lssq(i))),  + 0,  + 0,  + 0,  + (0 - (Lmq(i)^2*Lssq(i) + Lkq2(i)*Lkq3(i)*Lssq(i) - Lkq2(i)*Lmq(i)*Lssq(i) - Lkq3(i)*Lmq(i)*Lssq(i))/(3*Lmq(i)^4 - 2*Lkq2(i)*Lmq(i)^3 - 2*Lkq3(i)*Lmq(i)^3 - 2*Lmq(i)^3*Lssq(i) - 2*Lkq1(i)*Lmq(i)^3 + Lkq1(i)*Lkq2(i)*Lmq(i)^2 + Lkq1(i)*Lkq3(i)*Lmq(i)^2 + Lkq2(i)*Lkq3(i)*Lmq(i)^2 + Lkq1(i)*Lmq(i)^2*Lssq(i) + Lkq2(i)*Lmq(i)^2*Lssq(i) + Lkq3(i)*Lmq(i)^2*Lssq(i) - Lkq1(i)*Lkq2(i)*Lkq3(i)*Lssq(i))),  + 0,  + 0, ; 0,  + (0 + (Lmq(i)*(Lkq1(i) - Lmq(i))*(Lkq3(i) - Lmq(i)))/(3*Lmq(i)^4 - 2*Lkq2(i)*Lmq(i)^3 - 2*Lkq3(i)*Lmq(i)^3 - 2*Lmq(i)^3*Lssq(i) - 2*Lkq1(i)*Lmq(i)^3 + Lkq1(i)*Lkq2(i)*Lmq(i)^2 + Lkq1(i)*Lkq3(i)*Lmq(i)^2 + Lkq2(i)*Lkq3(i)*Lmq(i)^2 + Lkq1(i)*Lmq(i)^2*Lssq(i) + Lkq2(i)*Lmq(i)^2*Lssq(i) + Lkq3(i)*Lmq(i)^2*Lssq(i) - Lkq1(i)*Lkq2(i)*Lkq3(i)*Lssq(i))),  + 0,  + 0,  + 0,  + (0 - (Lssq(i)*(Lkq1(i) - Lmq(i))*(Lkq3(i) - Lmq(i)))/(3*Lmq(i)^4 - 2*Lkq2(i)*Lmq(i)^3 - 2*Lkq3(i)*Lmq(i)^3 - 2*Lmq(i)^3*Lssq(i) - 2*Lkq1(i)*Lmq(i)^3 + Lkq1(i)*Lkq2(i)*Lmq(i)^2 + Lkq1(i)*Lkq3(i)*Lmq(i)^2 + Lkq2(i)*Lkq3(i)*Lmq(i)^2 + Lkq1(i)*Lmq(i)^2*Lssq(i) + Lkq2(i)*Lmq(i)^2*Lssq(i) + Lkq3(i)*Lmq(i)^2*Lssq(i) - Lkq1(i)*Lkq2(i)*Lkq3(i)*Lssq(i))),  + 0,  + 0, ; 0,  + (0 + (Lmq(i)*(Lkq1(i) - Lmq(i))*(Lkq2(i) - Lmq(i)))/(3*Lmq(i)^4 - 2*Lkq2(i)*Lmq(i)^3 - 2*Lkq3(i)*Lmq(i)^3 - 2*Lmq(i)^3*Lssq(i) - 2*Lkq1(i)*Lmq(i)^3 + Lkq1(i)*Lkq2(i)*Lmq(i)^2 + Lkq1(i)*Lkq3(i)*Lmq(i)^2 + Lkq2(i)*Lkq3(i)*Lmq(i)^2 + Lkq1(i)*Lmq(i)^2*Lssq(i) + Lkq2(i)*Lmq(i)^2*Lssq(i) + Lkq3(i)*Lmq(i)^2*Lssq(i) - Lkq1(i)*Lkq2(i)*Lkq3(i)*Lssq(i))),  + 0,  + 0,  + 0,  + (0 - (Lssq(i)*(Lkq1(i) - Lmq(i))*(Lkq2(i) - Lmq(i)))/(3*Lmq(i)^4 - 2*Lkq2(i)*Lmq(i)^3 - 2*Lkq3(i)*Lmq(i)^3 - 2*Lmq(i)^3*Lssq(i) - 2*Lkq1(i)*Lmq(i)^3 + Lkq1(i)*Lkq2(i)*Lmq(i)^2 + Lkq1(i)*Lkq3(i)*Lmq(i)^2 + Lkq2(i)*Lkq3(i)*Lmq(i)^2 + Lkq1(i)*Lmq(i)^2*Lssq(i) + Lkq2(i)*Lmq(i)^2*Lssq(i) + Lkq3(i)*Lmq(i)^2*Lssq(i) - Lkq1(i)*Lkq2(i)*Lkq3(i)*Lssq(i))),  + 0,  + 0, ];
      |     end
  isd : Outport
  isq : Outport  Port=2
  psi : Outport  Port=3
  ifd : Outport  Port=4

== system AC_gen_MGES/MGES/For Each Subsystem ==
  In1 : Inport  Partition=on  PartitionDimension=1  PartitionWidth=1  PartitionOffset=0
  For Each : ForEach  DisableCoverage=on
  State-Space : StateSpace  A=[]  B=[]  C=[]  D=block_toM  InitialCondition=0  ParameterTunability=Optimized
  Transpose : Math  Operator=transpose
  Transpose1 : Math  Operator=transpose
  Out1 : Outport  ConcatenationDimension=1
  wires:
  State-Space/1 -> Transpose1/1
  Transpose/1 -> State-Space/1
  In1/1 -> Transpose/1
  Transpose1/1 -> Out1/1

== system AC_gen_MGES/MGES/LPF1 ==
  in : Inport
  Gain : Gain  Gain=1./T_s
  Sum4 : Sum  Inputs=|+-
  x_a : Integrator  InitialConditionSource=external  InitialCondition=Grid_op_MGES.op.States(16).x'
  out : Outport
  wires:
  x_a/1 -> Sum4/2, out/1
  in/1 -> Sum4/1, x_a/2
  Sum4/1 -> Gain/1
  Gain/1 -> x_a/1

== system AC_gen_MGES/MGES/LPF2 ==
  in : Inport
  Gain : Gain  Gain=1./T_s
  Sum4 : Sum  Inputs=|+-
  x_a : Integrator  InitialConditionSource=external  InitialCondition=Grid_op_MGES.op.States(17).x'
  out : Outport
  wires:
  x_a/1 -> Sum4/2, out/1
  in/1 -> Sum4/1, x_a/2
  Sum4/1 -> Gain/1
  Gain/1 -> x_a/1

== system AC_gen_MGES/MGES/LPF3 ==
  in : Inport
  Gain : Gain  Gain=1./T_s
  Sum4 : Sum  Inputs=|+-
  x_a : Integrator  InitialConditionSource=external  InitialCondition=Grid_op_MGES.op.States(18).x'
  out : Outport
  wires:
  x_a/1 -> Sum4/2, out/1
  in/1 -> Sum4/1, x_a/2
  Sum4/1 -> Gain/1
  Gain/1 -> x_a/1

== system AC_gen_MGES/MGES/LPF4 ==
  in : Inport
  Gain : Gain  Gain=1./T_s
  Sum4 : Sum  Inputs=|+-
  x_a : Integrator  InitialCondition=Grid_op_SG.op.States(10).x'
  out : Outport
  wires:
  Gain/1 -> x_a/1
  Sum4/1 -> Gain/1
  in/1 -> Sum4/1
  x_a/1 -> out/1, Sum4/2

== system AC_gen_MGES/MGES/LPF5 ==
  in : Inport
  Gain : Gain  Gain=1./T_s
  Sum4 : Sum  Inputs=|+-
  x_a : Integrator  InitialCondition=Grid_op_SG.op.States(11).x'
  out : Outport
  wires:
  x_a/1 -> Sum4/2, out/1
  in/1 -> Sum4/1
  Sum4/1 -> Gain/1
  Gain/1 -> x_a/1

== system AC_gen_MGES/MGES/LPF6 ==
  in : Inport
  Gain : Gain  Gain=1./T_s
  Sum4 : Sum  Inputs=|+-
  x_a : Integrator  InitialConditionSource=external  InitialCondition=Grid_op_MGES.op.States(19).x'
  out : Outport
  wires:
  x_a/1 -> Sum4/2, out/1
  in/1 -> Sum4/1, x_a/2
  Sum4/1 -> Gain/1
  Gain/1 -> x_a/1

== system AC_gen_MGES/MGES/LeadLag ==
  In1 : Inport
  AVR_LeadLag : Subsystem  mask{T_2=T_2(T_1~=0), T_1=T_1(T_1~=0)}
      mask help:
      | Transfer function:
      |
      |   1 + sT_2
      | ---------------
      |   1 + sT_1
  Assignment1 : Assignment  DiagnosticForDimensions=Warning  IndexOptions=Index vector (dialog)  Indices=find(T_1~=0)  OutputSizes=1
  Selector10 : Selector  InputPortWidth=length(block_buses)  IndexOptions=Index vector (dialog)  Indices=find(T_1~=0)  OutputSizes=1
  Out1 : Outport
  wires:
  In1/1 -> Selector10/1, Assignment1/1
  Assignment1/1 -> Out1/1
  Selector10/1 -> AVR_LeadLag/1(In1)
  AVR_LeadLag/1(Out1) -> Assignment1/2

== system AC_gen_MGES/MGES/LeadLag1 ==
  In1 : Inport
  Gain : Gain  Gain=1./T_1
  Gain2 : Gain  Gain=T_2./T_1
  Sum : Sum  Inputs=|+-
  Sum1 : Sum  Inputs=++|
  x_f : Integrator  InitialConditionSource=external  InitialCondition=Grid_op_MGES.op.States(21).x'
  Out1 : Outport
  wires:
  In1/1 -> Sum/1, x_f/2
  Sum1/1 -> Out1/1
  Gain2/1 -> Sum1/1
  Sum/1 -> Gain2/1, Gain/1
  Gain/1 -> x_f/1
  x_f/1 -> Sum/2, Sum1/2

== system AC_gen_MGES/MGES/LeadLag2 ==
  In1 : Inport
  Gain : Gain  Gain=1./T_1
  Gain2 : Gain  Gain=T_2./T_1
  Sum : Sum  Inputs=|+-
  Sum1 : Sum  Inputs=++|
  x_f : Integrator  InitialConditionSource=external  InitialCondition=Grid_op_MGES.op.States(22).x'
  Out1 : Outport
  wires:
  x_f/1 -> Sum1/2, Sum/2
  Gain/1 -> x_f/1
  Sum/1 -> Gain/1, Gain2/1
  Gain2/1 -> Sum1/1
  Sum1/1 -> Out1/1
  In1/1 -> x_f/2, Sum/1

== system AC_gen_MGES/MGES/PI1 ==
  In1 : Inport
  Gain1 : Gain  Gain=K_IM ~= 0
  Gain4 : Gain  Gain=K_PM
  Gain5 : Gain  Gain=K_IM
  Integrator : Integrator  InitialCondition=Grid_op_MGES.op.States(23).x'
  Sum7 : Sum  Inputs=|++
  vfd : Outport
  wires:
  Gain1/1 -> Sum7/2
  Gain5/1 -> Integrator/1
  In1/1 -> Gain5/1, Gain4/1
  Sum7/1 -> vfd/1
  Gain4/1 -> Sum7/1
  Integrator/1 -> Gain1/1

== system AC_gen_MGES/MGES/PI2 ==
  In1 : Inport
  Gain1 : Gain  Gain=K_IR ~= 0
  Gain4 : Gain  Gain=K_PR
  Gain5 : Gain  Gain=K_IR
  Integrator : Integrator  InitialCondition=Grid_op_MGES.op.States(24).x'
  Sum7 : Sum  Inputs=|++
  Out1 : Outport
  wires:
  Gain1/1 -> Sum7/2
  Gain5/1 -> Integrator/1
  In1/1 -> Gain5/1, Gain4/1
  Sum7/1 -> Out1/1
  Gain4/1 -> Sum7/1
  Integrator/1 -> Gain1/1

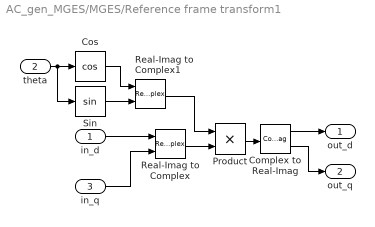
== system AC_gen_MGES/MGES/Reference frame transform1 ==
  in_d : Inport
  theta : Inport  Port=2
  in_q : Inport  Port=3
  Complex to Real-Imag : ComplexToRealImag
  Cos : Trigonometry  SCDEnableBlockLinearizationSpecification=on  Operator=cos
  Product : Product
  Real-Imag to Complex : RealImagToComplex
  Real-Imag to Complex1 : RealImagToComplex
  Sin : Trigonometry  SCDEnableBlockLinearizationSpecification=on
  out_d : Outport
  out_q : Outport  Port=2
  wires:
  Complex to Real-Imag/2 -> out_q/1
  Real-Imag to Complex1/1 -> Product/1
  Real-Imag to Complex/1 -> Product/2
  Product/1 -> Complex to Real-Imag/1
  theta/1 -> Sin/1, Cos/1
  Cos/1 -> Real-Imag to Complex1/1
  Sin/1 -> Real-Imag to Complex1/2
  Complex to Real-Imag/1 -> out_d/1
  in_q/1 -> Real-Imag to Complex/2
  in_d/1 -> Real-Imag to Complex/1

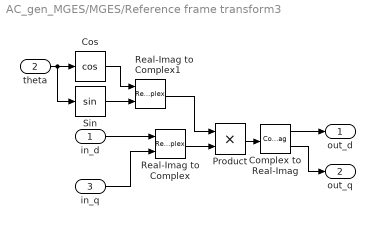
== system AC_gen_MGES/MGES/Reference frame transform3 ==
  in_d : Inport
  theta : Inport  Port=2
  in_q : Inport  Port=3
  Complex to Real-Imag : ComplexToRealImag
  Cos : Trigonometry  SCDEnableBlockLinearizationSpecification=on  Operator=cos
  Product : Product
  Real-Imag to Complex : RealImagToComplex
  Real-Imag to Complex1 : RealImagToComplex
  Sin : Trigonometry  SCDEnableBlockLinearizationSpecification=on
  out_d : Outport
  out_q : Outport  Port=2
  wires:
  in_d/1 -> Real-Imag to Complex/1
  in_q/1 -> Real-Imag to Complex/2
  Complex to Real-Imag/1 -> out_d/1
  Sin/1 -> Real-Imag to Complex1/2
  Cos/1 -> Real-Imag to Complex1/1
  theta/1 -> Cos/1, Sin/1
  Product/1 -> Complex to Real-Imag/1
  Real-Imag to Complex/1 -> Product/2
  Real-Imag to Complex1/1 -> Product/1
  Complex to Real-Imag/2 -> out_q/1

== system AC_gen_MGES/MGES/Rotor axis ==
  te : Inport
  tm : Inport  Port=2
  Gain : Gain  Gain=1/2./H
  Gain1 : Gain  Gain=D
  Sum1 : Sum  Inputs=+|-|-  InputSameDT=on  SaturateOnIntegerOverflow=on  OutDataTypeStr=Inherit: Same as first input
  \omega_r : Integrator  InitialCondition=Grid_op_MGES.op.States(25).x'  UpperSaturationLimit=2*pi  LowerSaturationLimit=0
  wr : Outport  VectorParamsAs1DForOutWhenUnconnected=off
  wires:
  Gain1/1 -> Sum1/3
  Gain/1 -> \omega_r/1
  Sum1/1 -> Gain/1
  te/1 -> Sum1/2
  \omega_r/1 -> Gain1/1, wr/1
  tm/1 -> Sum1/1

== system AC_gen_MGES/MGES/Subsystem ==
  in : Inport
  LPF1 : Subsystem  mask{T_s=T_9}
      mask prompts: T_s "Filter time constant"
  LPF2 : Subsystem  mask{T_s=T_9}
      mask prompts: T_s "Filter time constant"
  LPF3 : Subsystem  mask{T_s=T_9}
      mask prompts: T_s "Filter time constant"
  LPF4 : Subsystem  mask{T_s=T_9}
      mask prompts: T_s "Filter time constant"
  LPF7 : Subsystem  mask{T_s=T_9}
      mask prompts: T_s "Filter time constant"
  out : Outport
  wires:
  in/1 -> LPF7/1(in)
  LPF1/1(out) -> LPF2/1(in)
  LPF4/1(out) -> out/1
  LPF7/1(out) -> LPF1/1(in)
  LPF3/1(out) -> LPF4/1(in)
  LPF2/1(out) -> LPF3/1(in)

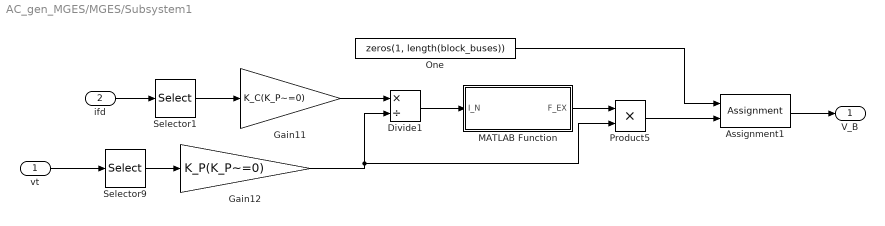
== system AC_gen_MGES/MGES/Subsystem1 ==
  vt : Inport
  ifd : Inport  Port=2
  Assignment1 : Assignment  DiagnosticForDimensions=Warning  IndexOptions=Index vector (dialog)  Indices=find(K_P~=0)  OutputSizes=1
  Divide1 : Product  Inputs=*/
  Gain11 : Gain  Gain=K_C(K_P~=0)
  Gain12 : Gain  Gain=K_P(K_P~=0)
  MATLAB Function : MATLAB Function  TreatAsAtomicUnit=on
  One : Constant  Value=zeros(1, length(block_buses))  VectorParams1D=off  OutDataTypeStr=Inherit: Inherit via back propagation
  Product5 : Product
  Selector1 : Selector  InputPortWidth=length(block_buses)  IndexOptions=Index vector (dialog)  Indices=find(K_P~=0)  OutputSizes=1
  Selector9 : Selector  InputPortWidth=length(block_buses)  IndexOptions=Index vector (dialog)  Indices=find(K_P~=0)  OutputSizes=1
  V_B : Outport
  wires:
  Divide1/1 -> MATLAB Function/1(I_N)
  Selector1/1 -> Gain11/1
  ifd/1 -> Selector1/1
  Gain12/1 -> Product5/2, Divide1/2
  MATLAB Function/1(F_EX) -> Product5/1
  Gain11/1 -> Divide1/1
  Selector9/1 -> Gain12/1
  Assignment1/1 -> V_B/1
  vt/1 -> Selector9/1
  One/1 -> Assignment1/1
  Product5/1 -> Assignment1/2

== system AC_gen_MGES/MGES/Subsystem4 ==
  In1 : Inport
  Gain : Gain  Gain=1./T_1
  Gain2 : Gain  Gain=T_2./T_1
  Sum : Sum  Inputs=|+-
  Sum1 : Sum  Inputs=++|
  x_f : Integrator  InitialCondition=Grid_op_MGES.op.States(21).x'
  Out1 : Outport
  wires:
  In1/1 -> Sum/1
  Sum1/1 -> Out1/1
  Gain2/1 -> Sum1/1
  Sum/1 -> Gain2/1, Gain/1
  Gain/1 -> x_f/1
  x_f/1 -> Sum/2, Sum1/2

== system AC_gen_MGES/MGES/Torque ==
  psi : Inport
  isd : Inport  Port=2
  isq : Inport  Port=3
  Product1 : Product
  Product2 : Product
  Selector : Selector  NumberOfDimensions=2  InputPortWidth=9  IndexOptions=Index vector (dialog),Select all  Indices=[1],1  OutputSizes=1,1
  Selector1 : Selector  NumberOfDimensions=2  InputPortWidth=9  IndexOptions=Index vector (dialog),Select all  Indices=[2],1  OutputSizes=1,1
  Sum : Sum  Inputs=+||-
  te : Outport  VectorParamsAs1DForOutWhenUnconnected=off
  wires:
  Selector1/1 -> Product2/2  "psistatordq"
  isd/1 -> Product2/1
  isq/1 -> Product1/2
  Product2/1 -> Sum/2
  psi/1 -> Selector/1, Selector1/1
  Selector/1 -> Product1/1  "psistatordq"
  Sum/1 -> te/1
  Product1/1 -> Sum/1

== system AC_gen_MGES/MGES/WOF_d ==
  In1 : Inport
  Gain : Gain  Gain=1/T_w1
  I : Integrator  InitialConditionSource=external  InitialCondition=Grid_op_MGES.op.States(31).x'
  Sum : Sum  Inputs=+-|
  Sum4 : Sum  Inputs=|+-
  Out1 : Outport
  wires:
  Gain/1 -> I/1
  Sum4/1 -> Gain/1
  In1/1 -> I/2, Sum/1, Sum4/1
  I/1 -> Sum4/2, Sum/2
  Sum/1 -> Out1/1

== system AC_gen_MGES/MGES/WOF_d1 ==
  In1 : Inport
  Gain : Gain  Gain=1/T_w2
  I : Integrator  InitialConditionSource=external  InitialCondition=Grid_op_MGES.op.States(32).x'
  Sum : Sum  Inputs=+-|
  Sum4 : Sum  Inputs=|+-
  Out1 : Outport
  wires:
  Gain/1 -> I/1
  Sum4/1 -> Gain/1
  In1/1 -> I/2, Sum/1, Sum4/1
  I/1 -> Sum4/2, Sum/2
  Sum/1 -> Out1/1

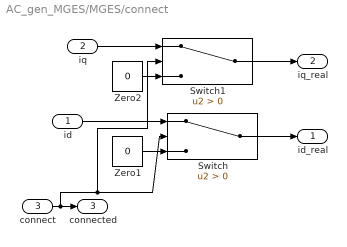
== system AC_gen_MGES/MGES/connect ==
  id : Inport
  iq : Inport  Port=2
  connect : Inport  Port=3
  Switch : Switch  Criteria=u2 > Threshold  ZeroCross=off  SaturateOnIntegerOverflow=off  InputSameDT=off
  Switch1 : Switch  Criteria=u2 > Threshold  ZeroCross=off  SaturateOnIntegerOverflow=off  InputSameDT=off
  Zero1 : Constant  Value=0  VectorParams1D=off  OutDataTypeStr=Inherit: Inherit via back propagation
  Zero2 : Constant  Value=0  VectorParams1D=off  OutDataTypeStr=Inherit: Inherit via back propagation
  id_real : Outport
  iq_real : Outport  Port=2
  connected : Outport  Port=3  OutDataTypeStr=boolean
  wires:
  Zero2/1 -> Switch1/3
  iq/1 -> Switch1/1
  Switch1/1 -> iq_real/1
  connect/1 -> Switch/2, Switch1/2, connected/1
  id/1 -> Switch/1
  Zero1/1 -> Switch/3
  Switch/1 -> id_real/1

== system AC_gen_MGES/MGES/trim_output ==
  id : Inport
  iq : Inport  Port=2
  vd : Inport  Port=3
  vq : Inport  Port=4
  Out1 : Outport
  Out2 : Outport  Port=2
  Out3 : Outport  Port=3
  Out4 : Outport  Port=4
  wires:
  iq/1 -> Out2/1
  vd/1 -> Out3/1
  vq/1 -> Out4/1
  id/1 -> Out1/1

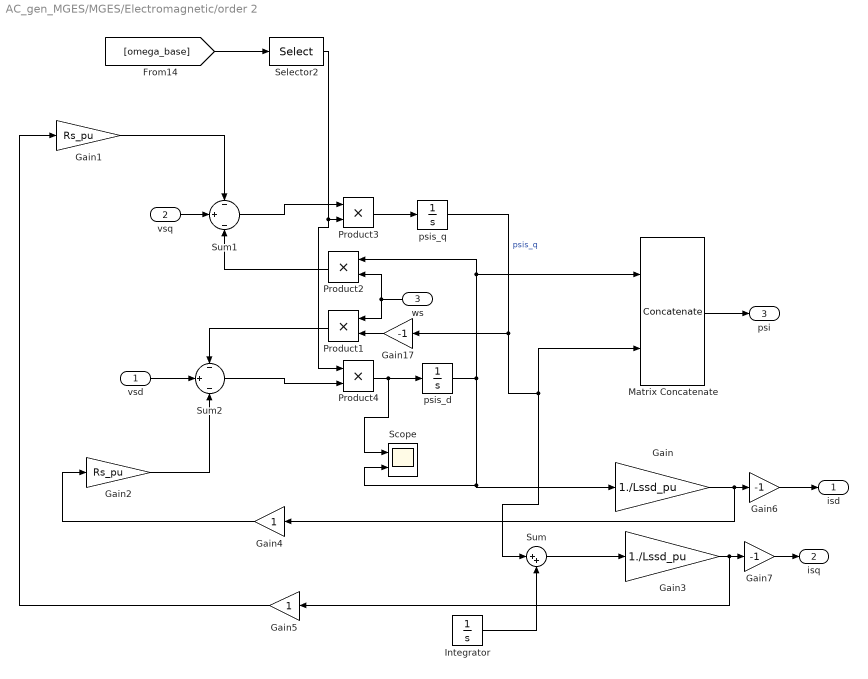
== system AC_gen_MGES/MGES/Electromagnetic/order 2 ==
  vsd : Inport
  vsq : Inport  Port=2
  ws : Inport  Port=3
  Gain : Gain  Gain=1./Lssd_pu
  Gain1 : Gain  Gain=Rs_pu
  Gain17 : Gain  Gain=-1
  Gain2 : Gain  Gain=Rs_pu
  Gain3 : Gain  Gain=1./Lssd_pu
  Gain4 : Gain
  Gain5 : Gain
  Gain6 : Gain  Gain=-1
  Gain7 : Gain  Gain=-1
  Integrator : Integrator  InitialCondition=Grid_op_MGES.op.States(5).x'
  Matrix Concatenate : Concatenate  Mode=Multidimensional array
  Product{1..4} (4 alike) : Product
  Scope : Scope  NumInputPorts=2
      settings: ActiveDisplayYMinimum=-176.647  ActiveDisplayYMaximum=19.6557
  Selector2 : Selector  InputPortWidth=length(fref.ref_units)  IndexOptions=Index vector (dialog)  Indices=block_fref  OutputSizes=1
  Sum : Sum  Inputs=|++
  Sum1 : Sum  Inputs=-|+|-  InputSameDT=on  SaturateOnIntegerOverflow=on  OutDataTypeStr=Inherit: Same as first input
  Sum2 : Sum  Inputs=-|+|-  InputSameDT=on  SaturateOnIntegerOverflow=on  OutDataTypeStr=Inherit: Same as first input
  psis_d : Integrator  InitialCondition=Grid_op_MGES.op.States(6).x'
  psis_q : Integrator  InitialCondition=Grid_op_MGES.op.States(7).x'
  isd : Outport  VectorParamsAs1DForOutWhenUnconnected=off
  isq : Outport  Port=2  VectorParamsAs1DForOutWhenUnconnected=off
  psi : Outport  Port=3  VectorParamsAs1DForOutWhenUnconnected=off
  wires:
  Gain7/1 -> isq/1
  Gain6/1 -> isd/1
  psis_d/1 -> Scope/2, Gain/1, Matrix Concatenate/1, Product2/1
  Gain5/1 -> Gain1/1
  Gain4/1 -> Gain2/1
  Integrator/1 -> Sum/2
  Sum/1 -> Gain3/1
  Selector2/1 -> Product3/2, Product4/1
  Gain17/1 -> Product1/2
  Gain3/1 -> Gain7/1, Gain5/1
  Gain2/1 -> Sum2/3
  Gain/1 -> Gain6/1, Gain4/1
  vsq/1 -> Sum1/2
  [omega_base] -> Selector2/1
  Gain1/1 -> Sum1/1
  psis_q/1 -> Gain17/1, Matrix Concatenate/2, Sum/1  "psis_q"
  Sum2/1 -> Product4/2
  Product2/1 -> Sum1/3
  Product1/1 -> Sum2/1
  Sum1/1 -> Product3/1
  Product3/1 -> psis_q/1
  Matrix Concatenate/1 -> psi/1
  ws/1 -> Product2/2, Product1/1
  vsd/1 -> Sum2/2
  Product4/1 -> psis_d/1, Scope/1

== system AC_gen_MGES/MGES/Electromagnetic/order 8 ==
  vsd : Inport
  vsq : Inport  Port=2
  vfd : Inport  Port=3
  ws : Inport  Port=4
  Stator circuit : Subsystem
  psi->i : Subsystem
  isd : Outport
  isq : Outport  Port=2
  psi : Outport  Port=3
  ifd : Outport  Port=4
  wires:
  psi->i/4(ifd) -> ifd/1
  psi->i/1(isd) -> isd/1
  vfd/1 -> Stator circuit/5(vfd)
  Stator circuit/1(psi) -> psi->i/1(psi), psi/1
  ws/1 -> Stator circuit/4(ws)
  vsq/1 -> Stator circuit/2(vsq)
  vsd/1 -> Stator circuit/1(vsd)
  psi->i/2(i) -> Stator circuit/3(i)
  psi->i/3(isq) -> isq/1

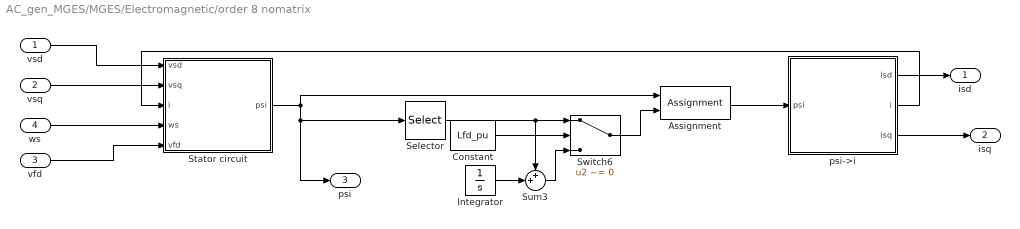
== system AC_gen_MGES/MGES/Electromagnetic/order 8 nomatrix ==
  vsd : Inport
  vsq : Inport  Port=2
  vfd : Inport  Port=3
  ws : Inport  Port=4
  Assignment : Assignment  NumberOfDimensions=2  DiagnosticForDimensions=Warning  IndexOptions=Index vector (dialog),Assign all  Indices=2,1  OutputSizes=1,1
  Constant : Constant  Value=Lfd_pu  VectorParams1D=off
  Integrator : Integrator  InitialCondition=Grid_op_MGES.op.States(5).x'
  Selector : Selector  NumberOfDimensions=2  InputPortWidth=3  IndexOptions=Index vector (dialog),Select all  Indices=2,1  OutputSizes=1,1
  Stator circuit : Subsystem
  Sum3 : Sum  Inputs=++|
  Switch6 : Switch  Criteria=u2 ~= 0  SaturateOnIntegerOverflow=off  InputSameDT=off
  psi->i : Subsystem
  isd : Outport
  isq : Outport  Port=2
  psi : Outport  Port=3
  wires:
  Switch6/1 -> Assignment/2
  Selector/1 -> Switch6/1, Sum3/1
  Assignment/1 -> psi->i/1(psi)
  Integrator/1 -> Sum3/2
  Constant/1 -> Switch6/2
  Sum3/1 -> Switch6/3
  psi->i/1(isd) -> isd/1
  vfd/1 -> Stator circuit/5(vfd)
  Stator circuit/1(psi) -> Assignment/1, Selector/1, psi/1
  ws/1 -> Stator circuit/4(ws)
  vsq/1 -> Stator circuit/2(vsq)
  vsd/1 -> Stator circuit/1(vsd)
  psi->i/2(i) -> Stator circuit/3(i)
  psi->i/3(isq) -> isq/1

== system AC_gen_MGES/MGES/LeadLag/AVR_LeadLag ==
  In1 : Inport
  Gain : Gain  Gain=1./T_1
  Gain2 : Gain  Gain=T_2./T_1
  Sum : Sum  Inputs=|+-
  Sum1 : Sum  Inputs=++|
  x_f : Integrator  InitialConditionSource=external  InitialCondition=Grid_op_MGES.op.States(20).x'
  Out1 : Outport
  wires:
  In1/1 -> Sum/1, x_f/2
  Sum1/1 -> Out1/1
  Gain2/1 -> Sum1/1
  Sum/1 -> Gain2/1, Gain/1
  Gain/1 -> x_f/1
  x_f/1 -> Sum/2, Sum1/2

== system AC_gen_MGES/MGES/Subsystem/LPF1 ==
  in : Inport
  Gain : Gain  Gain=1./T_s
  Sum4 : Sum  Inputs=|+-
  x_a : Integrator  InitialConditionSource=external  InitialCondition=Grid_op_MGES.op.States(26).x'
  out : Outport
  wires:
  Gain/1 -> x_a/1
  Sum4/1 -> Gain/1
  in/1 -> Sum4/1, x_a/2
  x_a/1 -> out/1, Sum4/2

== system AC_gen_MGES/MGES/Subsystem/LPF2 ==
  in : Inport
  Gain : Gain  Gain=1./T_s
  Sum4 : Sum  Inputs=|+-
  x_a : Integrator  InitialConditionSource=external  InitialCondition=Grid_op_MGES.op.States(27).x'
  out : Outport
  wires:
  Gain/1 -> x_a/1
  Sum4/1 -> Gain/1
  in/1 -> Sum4/1, x_a/2
  x_a/1 -> out/1, Sum4/2

== system AC_gen_MGES/MGES/Subsystem/LPF3 ==
  in : Inport
  Gain : Gain  Gain=1./T_s
  Sum4 : Sum  Inputs=|+-
  x_a : Integrator  InitialConditionSource=external  InitialCondition=Grid_op_MGES.op.States(28).x'
  out : Outport
  wires:
  Gain/1 -> x_a/1
  Sum4/1 -> Gain/1
  in/1 -> Sum4/1, x_a/2
  x_a/1 -> out/1, Sum4/2

== system AC_gen_MGES/MGES/Subsystem/LPF4 ==
  in : Inport
  Gain : Gain  Gain=1./T_s
  Sum4 : Sum  Inputs=|+-
  x_a : Integrator  InitialConditionSource=external  InitialCondition=Grid_op_MGES.op.States(29).x'
  out : Outport
  wires:
  Gain/1 -> x_a/1
  Sum4/1 -> Gain/1
  in/1 -> Sum4/1, x_a/2
  x_a/1 -> out/1, Sum4/2

== system AC_gen_MGES/MGES/Subsystem/LPF7 ==
  in : Inport
  Gain : Gain  Gain=1./T_s
  Sum4 : Sum  Inputs=|+-
  x_a : Integrator  InitialConditionSource=external  InitialCondition=Grid_op_MGES.op.States(30).x'
  out : Outport
  wires:
  Gain/1 -> x_a/1
  Sum4/1 -> Gain/1
  in/1 -> Sum4/1, x_a/2
  x_a/1 -> out/1, Sum4/2
